simulink model "AFSMC"  (R2013b)
settings: Solver=ode5  StartTime=0.0  StopTime=30  FixedStep=1e-4  RelTol=1e-3
undefined symbols (not defined in the file): A, B, beta, bm, Bp, C, DeltaA, DeltaB, H, K, L, x0
libraries: simulink x1
settings Model: Creator=oveisahw  LastModifiedBy=oveisahw

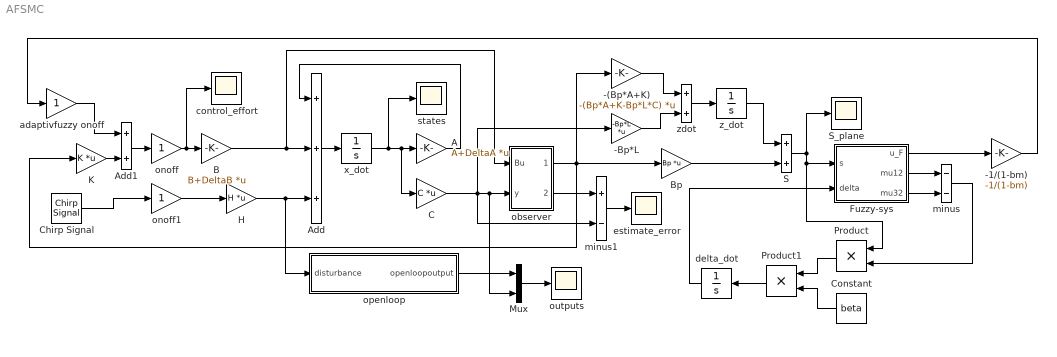
== system AFSMC ==
  -(Bp*A+K) : Gain  Gain=-(Bp*A+K-Bp*L*C)  Multiplication=Matrix(K*u) (u vector)
  -1/(1-bm) : Gain  Gain=-1/(1-bm)
  -Bp*L : Gain  Gain=-Bp*L  Multiplication=Matrix(K*u) (u vector)
  A : Gain  Gain=A+DeltaA  Multiplication=Matrix(K*u) (u vector)
  Add : Sum  Inputs=+++
  Add1 : Sum
  B : Gain  Gain=B+DeltaB  Multiplication=Matrix(K*u) (u vector)
  Bp : Gain  Gain=Bp  Multiplication=Matrix(K*u) (u vector)
  C : Gain  Gain=C  Multiplication=Matrix(K*u) (u vector)
  Chirp Signal : simulink/Sources/Chirp Signal  f1=0  T=30  f2=90
  Constant : Constant  Value=beta
  Fuzzy-sys : MATLAB Function  TreatAsAtomicUnit=on
  H : Gain  Gain=H  Multiplication=Matrix(K*u) (u vector)
  K : Gain  Gain=K  Multiplication=Matrix(K*u) (u vector)
  Mux : Mux  Inputs=2
  Product : Product
  Product1 : Product
  S : Sum
  S_plane : Scope
      settings: SaveName=ScopeData3
  adaptivfuzzy onoff : Gain
  control_effort : Scope
  delta_dot : Integrator
  estimate_error : Scope
  minus : Sum  Inputs=--
  minus1 : Sum  Inputs=+-
  observer : Subsystem
  onoff : Gain
  onoff1 : Gain
  openloop : Subsystem
  outputs : Scope
      settings: SaveName=ScopeData2
  states : Scope
      settings: SaveName=ScopeData4
  x_dot : Integrator
  z_dot : Integrator  InitialCondition=-Bp*x0
  zdot : Sum
  wires:
  H/1 -> openloop/1(disturbance), Add/3
  Chirp Signal/1 -> onoff1/1
  onoff1/1 -> H/1
  Add/1 -> x_dot/1
  x_dot/1 -> states/1, A/1, C/1
  A/1 -> Add/1
  C/1 -> -Bp*L/1, minus1/2, Mux/2, observer/2(y)
  observer/2(yhat) -> minus1/1
  minus1/1 -> estimate_error/1
  observer/1(xhat) -> K/1, -(Bp*A+K)/1, Bp/1
  Bp/1 -> S/2
  zdot/1 -> z_dot/1
  -(Bp*A+K)/1 -> zdot/1
  -Bp*L/1 -> zdot/2
  z_dot/1 -> S/1
  S/1 -> S_plane/1, Product/1, Fuzzy-sys/1(s)
  Fuzzy-sys/2(mu12) -> minus/1
  Fuzzy-sys/3(mu32) -> minus/2
  minus/1 -> Product/2
  Product/1 -> Product1/1
  Constant/1 -> Product1/2
  Product1/1 -> delta_dot/1
  delta_dot/1 -> Fuzzy-sys/2(delta)
  Fuzzy-sys/1(u_F) -> -1/(1-bm)/1
  K/1 -> Add1/2
  Add1/1 -> onoff/1
  onoff/1 -> control_effort/1, B/1
  B/1 -> observer/1(Bu), Add/2
  Mux/1 -> outputs/1
  openloop/1(openloopoutput) -> Mux/1
  adaptivfuzzy onoff/1 -> Add1/1
  -1/(1-bm)/1 -> adaptivfuzzy onoff/1

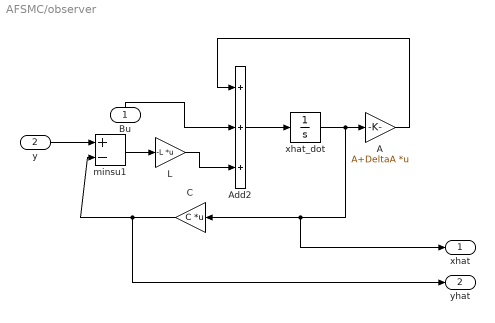
== system AFSMC/observer ==
  Bu : Inport
  y : Inport  Port=2
  A : Gain  Gain=A+DeltaA  Multiplication=Matrix(K*u) (u vector)
  Add2 : Sum  Inputs=+++
  C : Gain  Gain=C  Multiplication=Matrix(K*u) (u vector)
  L : Gain  Gain=-L  Multiplication=Matrix(K*u) (u vector)
  minsu1 : Sum  Inputs=+-
  xhat_dot : Integrator
  xhat : Outport
  yhat : Outport  Port=2
  wires:
  A/1 -> Add2/1
  L/1 -> Add2/3
  minsu1/1 -> L/1
  Add2/1 -> xhat_dot/1
  y/1 -> minsu1/1
  xhat_dot/1 -> xhat/1, C/1, A/1
  C/1 -> yhat/1, minsu1/2
  Bu/1 -> Add2/2

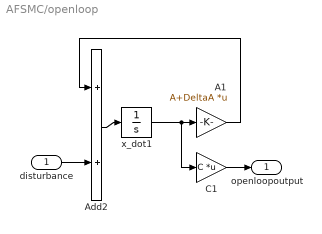
== system AFSMC/openloop ==
  disturbance : Inport
  A1 : Gain  Gain=A+DeltaA  Multiplication=Matrix(K*u) (u vector)
  Add2 : Sum
  C1 : Gain  Gain=C  Multiplication=Matrix(K*u) (u vector)
  x_dot1 : Integrator
  openloopoutput : Outport
  wires:
  disturbance/1 -> Add2/2
  x_dot1/1 -> A1/1, C1/1
  Add2/1 -> x_dot1/1
  A1/1 -> Add2/1
  C1/1 -> openloopoutput/1

== matlab function AFSMC/Fuzzy-sys ==
  data: s input; u_F output; delta input; mu12 output; mu32 output
function [u_F,mu12,mu32] = fcn(s,delta)
%#codegen
u = s;
m = 2;
a = 0.1;
mu12 = zeros(m,1);
mu32 = zeros(m,1);
for i = 1:m
    y = zeros(m,1);
    if u(i,1) <= -a
        mu1 = 1;
        mu2 = 0;
        mu3 = 0;
    elseif -a < u(i,1) && u(i,1) <= 0
        mu1 = -1/a*u(i,1);
        mu2 = 1/a*(u(i,1)+a);
        mu3 = 0;
    elseif a >= u(i,1) && u(i,1) > 0
        mu1 = 0;
        mu2 = -1/a*(u(i,1)-a);
        mu3 = 1/a*u(i,1);
    elseif u(i,1) > a
        mu1 = 0;
        mu2 = 0;
        mu3 = 1;
    else
        mu1 = 1000;
        mu2 = 1000;
        mu3 = 1000;
    end

    mu12(i,1) = mu1;
    mu32(i,1) = mu3;
    y(i,1) = (mu1*(-delta(i,1))+mu2*0+mu3*delta(i,1))/(mu1+mu2+mu3);
end
u_F = y;
